simulink model "descent_model"  (R2013a)
settings: Solver=ode45  StartTime=0.0  StopTime=t_stop  RelTol=1e-5
values from neighbouring files (symbols this model uses):
  A = pi * (6/2)^2 * 0.092903    (= 2.62677044067)    [hab6_55.m]
  alt0 = alt_1    [hab6_55.m]
  CD = CD_vec(q)    [hab6_55.m]
  m = 15 * 0.453592    (= 6.80388)    [hab6_55.m]
  v0 = v0_1    [hab6_55.m]
settings Model: Creator=justiceb  LastModifiedBy=Willdog
settings DebuggingCC: SolverPrmCheckMsg=none

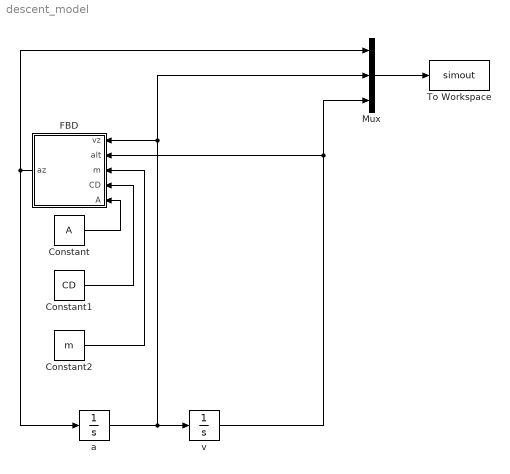
== system descent_model ==
  Constant : Constant  Value=A
  Constant1 : Constant  Value=CD
  Constant2 : Constant  Value=m
  FBD : MATLAB Function  TreatAsAtomicUnit=on
  Mux : Mux  Inputs=3
  To Workspace : ToWorkspace  VariableName=simout  SampleTime=-1  SaveFormat=Timeseries
  a : Integrator  InitialCondition=v0
  v : Integrator  InitialCondition=alt0
  wires:
  a/1 -> v/1, FBD/1(vz), Mux/2
  FBD/1(az) -> a/1, Mux/1
  Mux/1 -> To Workspace/1
  v/1 -> Mux/3, FBD/2(alt)
  Constant2/1 -> FBD/3(m)
  Constant1/1 -> FBD/4(CD)
  Constant/1 -> FBD/5(A)

== matlab function descent_model/FBD ==
  data: vz input; az output; alt input; m input; CD input; A input
function az = fcn(vz,alt,m,CD,A)

% must declare as extrinsic so that is runs in matlab environment
coder.extrinsic('stdatmo');

% Find air density at this altitude
rho_air = 0;                             %define to be a double
[rho_air,sos,T,P,nu,ZorH]=stdatmo(alt);  %SI  (standard atmosphere)

%calculate net acceleration
az = (0.5 * rho_air * vz^2 * A * CD)/m - 9.81;

end
